simulink model "ICL2L"  (R2021a)
settings: Solver=ode1  StartTime=0.0  StopTime=30.0  FixedStep=P.ts  RelTol=1e-3  EnableMultiTasking=on
InitFcn:
  | ICL2L_PreSim
undefined symbols (not defined in the file or in its folder): P
libraries: commchan3 x2, commfilt2 x2
settings Model: Creator=rkamalapurkar  LastModifiedBy=rushik
settings SolverCC: AlgebraicLoopSolver=TrustRegion
settings DataIOCC: LimitDataPoints=on  SaveFormat=Array  SignalLoggingSaveFormat=ModelDataLogs  ReturnWorkspaceOutputs=off
settings OptimizationCC: ExpressionDepthLimit=2147483647  LifeSpan=inf
settings DebuggingCC: UnderspecifiedInitializationDetection=Classic  MergeDetectMultiDrivingBlocksExec=none  SolverPrmCheckMsg=warning  FcnCallInpInsideContextMsg=warning  StateNameClashWarn=warning  SFUnexpectedBacktrackingDiag=warning  SFNoUnconditionalDefaultTransitionDiag=warning  SFExecutionAtInitializationDiag=none  SFMachineParentedDataDiag=warning  ArithmeticOperatorsInVariantConditions=warning
settings HardwareCC: ProdBitPerPointer=32  ProdBitPerSizeT=32  ProdBitPerPtrDiffT=32  ProdLargestAtomicFloat=None  ProdIntDivRoundTo=Undefined  ProdEndianess=Unspecified  ProdWordSize=32  ProdHWDeviceType=32-bit Generic
settings ModelReferenceCC: PropagateSignalLabelsOutOfModel=off
settings SFSimCC: SimUseLocalCustomCode=off  CustomCodeUndefinedFunction=UseInterfaceOnly
settings RTWCC: RTWUseLocalCustomCode=off
settings CodeAppCC: StateflowObjectComments=on
settings GRTTargetCC: TargetLangStandard=C89/C90 (ANSI)  CombineOutputUpdateFcns=off  GRTInterface=on
settings ConfigComp: CovMetricSettings=dw  CovSaveCumulativeToWorkspaceVar=on  CovSaveSingleToWorkspaceVar=on  CovExternalEMLEnable=off  CovSFcnEnable=off

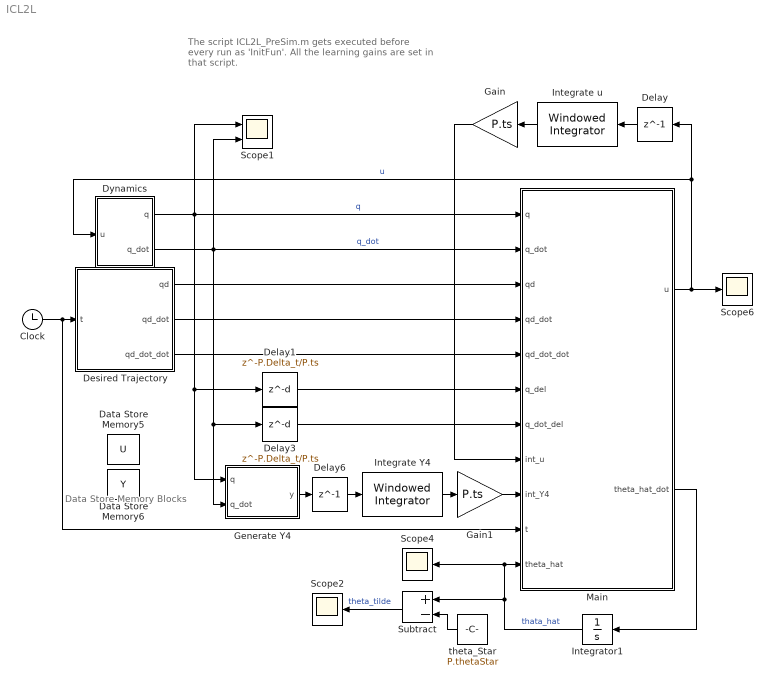
== system ICL2L ==
  note: Data Store Memory Blocks
  note: The script ICL2L_PreSim.m gets executed before every run as 'InitFun'. All the learning gains are set in that script.
  Clock : Clock
  Data Store Memory5 : DataStoreMemory  DataStoreName=U  InitialValue=zeros(P.n*P.N,1)  ShowAdditionalParam=off  OutDataTypeStr=double
  Data Store Memory6 : DataStoreMemory  DataStoreName=Y  InitialValue=zeros(P.n*P.N,P.L)  ShowAdditionalParam=off  OutDataTypeStr=double
  Delay : Delay  DelayLength=1
  Delay1 : Delay  DelayLength=P.Delta_t/P.ts  InitialCondition=0
  Delay3 : Delay  DelayLength=P.Delta_t/P.ts  InitialCondition=0
  Delay6 : Delay  DelayLength=1
  Desired Trajectory : MATLAB Function  TreatAsAtomicUnit=on
  Dynamics : Subsystem
  Gain : Gain  Gain=P.ts
  Gain1 : Gain  Gain=P.ts
  Generate Y4 : MATLAB Function  TreatAsAtomicUnit=on
  Integrate Y4 : commfilt2/Windowed Integrator  integperiod=P.Delta_t/P.ts  roundingMode=Floor  overflowMode=off  coeffDataTypeStr=Inherit: Same word length as input  coeffMin=[]  coeffMax=[]  coeffLastDataTypeStr=Inherit: Same word length as input  accumDataTypeStr=Inherit: Same as product output  accumLastDataTypeStr=Inherit: Same as product output  outputDataTypeStr=Inherit: Same as accumulator  outputMin=[]  outputMax=[]  outputLastDataTypeStr=Inherit: Same as accumulator
      settings: SourceProductBaseCode=CM
  Integrate u : commfilt2/Windowed Integrator  integperiod=P.Delta_t/P.ts  roundingMode=Floor  overflowMode=off  coeffDataTypeStr=Inherit: Same word length as input  coeffMin=[]  coeffMax=[]  coeffLastDataTypeStr=Inherit: Same word length as input  accumDataTypeStr=Inherit: Same as product output  accumLastDataTypeStr=Inherit: Same as product output  outputDataTypeStr=Inherit: Same as accumulator  outputMin=[]  outputMax=[]  outputLastDataTypeStr=Inherit: Same as accumulator
      settings: SourceProductBaseCode=CM
  Integrator1 : Integrator  InitialCondition=P.theta0
  Main : MATLAB Function  TreatAsAtomicUnit=on
  Scope1 : Scope  NumInputPorts=2
  Scope2 : Scope
  Scope4 : Scope
  Scope6 : Scope
  Subtract : Sum  Inputs=+-
  theta_Star : Constant  Value=P.thetaStar
  wires:
  Clock/1 -> Main/10(t), Desired Trajectory/1(t)
  Main/2(theta_hat_dot) -> Integrator1/1
  Integrator1/1 -> Scope4/1, Main/11(theta_hat), Subtract/1  "thata_hat"
  Dynamics/1(q) -> Scope1/1, Generate Y4/1(q), Delay1/1, Main/1(q)  "q"
  Main/1(u) -> Delay/1, Dynamics/1(u), Scope6/1  "u"
  Desired Trajectory/1(qd) -> Main/3(qd)
  Desired Trajectory/2(qd_dot) -> Main/4(qd_dot)
  Desired Trajectory/3(qd_dot_dot) -> Main/5(qd_dot_dot)
  Dynamics/2(q_dot) -> Scope1/2, Main/2(q_dot), Generate Y4/2(q_dot), Delay3/1  "q_dot"
  Delay3/1 -> Main/7(q_dot_del)
  Delay1/1 -> Main/6(q_del)
  Integrate u/1 -> Gain/1
  Gain/1 -> Main/8(int_u)
  Delay/1 -> Integrate u/1
  Integrate Y4/1 -> Gain1/1
  Gain1/1 -> Main/9(int_Y4)
  Generate Y4/1(y) -> Delay6/1
  Delay6/1 -> Integrate Y4/1
  Subtract/1 -> Scope2/1  "theta_tilde"
  theta_Star/1 -> Subtract/2

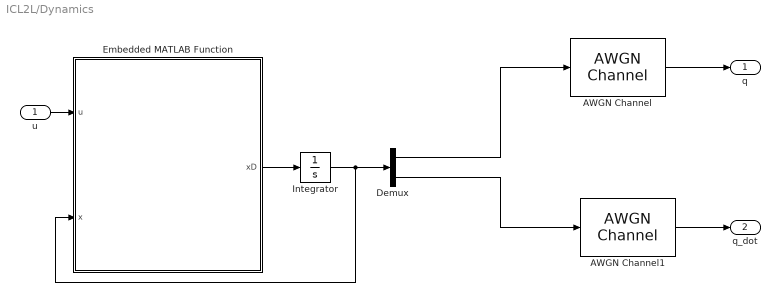
== system ICL2L/Dynamics ==
  u : Inport
  AWGN Channel : commchan3/AWGN Channel  InputProcessing=Columns as channels (frame based)  seed=67  noiseMode=Variance from mask  EbNodB=10  EsNodB=10  SNRdB=10  bitsPerSym=1  Ps=1  Tsym=1  variance=0.001
  AWGN Channel1 : commchan3/AWGN Channel  InputProcessing=Columns as channels (frame based)  seed=67  noiseMode=Variance from mask  EbNodB=10  EsNodB=10  SNRdB=10  bitsPerSym=1  Ps=1  Tsym=1  variance=0.01
  Demux : Demux  Outputs=2
  Embedded MATLAB Function : MATLAB Function  TreatAsAtomicUnit=on
  Integrator : Integrator  InitialCondition=P.x0
  q : Outport
  q_dot : Outport  Port=2
  wires:
  Integrator/1 -> Demux/1, Embedded MATLAB Function/2(x)
  Embedded MATLAB Function/1(xD) -> Integrator/1
  u/1 -> Embedded MATLAB Function/1(u)
  Demux/1 -> AWGN Channel/1
  Demux/2 -> AWGN Channel1/1
  AWGN Channel/1 -> q/1
  AWGN Channel1/1 -> q_dot/1

== matlab function ICL2L/Dynamics/Embedded MATLAB Function ==
  data: u input size=[P.n 1]; xD output size=[2*P.n 1]; x input size=[2*P.n 1]
function xD = fcn(u,x)

p1 = 3.473;
p2 = .196;
p3 = .242;
fd1 = 5.3;
fd2 = 1.1;
fs1 = 8.45;
fs2 = 2.35;

Minv = (1/(p2^2 - p1*p2 + p3^2*cos(x(2))^2))*...
       [-p2               p2+p3*cos(x(2))  ;...
         p2+p3*cos(x(2)) -p1-2*p3*cos(x(2))];

Vm = [-p3*sin(x(2))*x(4) -p3*sin(x(2))*(x(3)+x(4));
       p3*sin(x(2))*x(3)  0                      ];
Fd = diag([fd1,fd2]);
Fs = [fs1*tanh(1*x(3));fs2*tanh(1*x(4))];
f = [x(3); x(4); Minv*((-Vm - Fd)*[x(3); x(4)]-Fs)];
g = [0 0; 0 0; Minv]; 

xD = f+g*u;

== matlab function ICL2L/Generate Y4 ==
  data: q input size=[P.n 1]; y output size=[P.n P.L]; q_dot input size=[P.n 1]
function y = Y4(q,q_dot)
    y = Y4(q,q_dot);
end

== matlab function ICL2L/Desired Trajectory ==
  data: t input; qd output; qd_dot output; qd_dot_dot output
function [qd,qd_dot,qd_dot_dot] = desiredTrajectory(t)
    [qd,qd_dot,qd_dot_dot] = desiredTraj(t);
end

== matlab function ICL2L/Main ==
  settings: updateMethod=DISCRETE
  data: u output; q input size=[P.n 1]; q_dot input size=[P.n 1]; qd input; qd_dot input; qd_dot_dot input; q_del input; q_dot_del input; int_u input; int_Y4 input; t input; theta_hat input; theta_hat_dot output; U data_store_memory; P parameter; Y data_store_memory
function [u,theta_hat_dot] =...
    ICLControl(q,q_dot,qd,qd_dot,qd_dot_dot,q_del,q_dot_del,...
    int_u,int_Y4,t,theta_hat,P)
%#codegen
% This simulink block implements integral-concurrent-learning based system
% identification and adaptive control

global Y; % Data store memory for storing the values of \mathscr{Y}
          % nN x L
global U; % Data store memory for storing the values of \mathscr{U}
          % nN x 1
          
e = qd - q;
e_dot = qd_dot - q_dot;
r = e_dot + P.alpha * e;

if t > P.Delta_t
    % eigenvalue maximization data storage
    current_sum = Y.'*Y;
    current_min = min(eig(current_sum));
    new_Y = Y3(q,q_dot,q_del,q_dot_del) + int_Y4;
    new_U = int_u;
    min_store = zeros(P.N,1);
    for i=1:P.N
        new_sum = current_sum - Y(P.n*i-1:P.n*i,:).'*Y(P.n*i-1:P.n*i,:) + new_Y.'*new_Y;
        min_store(i) = real(min(eig(new_sum)));
    end
    [new_max,index] = max(min_store);
    if new_max > current_min + P.epsilon
            Y(P.n*index-1:P.n*index,:) = new_Y;
            U(P.n*index-1:P.n*index,:) = new_U;
    end

    % Update law
    theta_hat_dot = P.Gamma*Y2(q,q_dot,qd,qd_dot,qd_dot_dot,P.alpha).'*r...
        + P.k2*P.Gamma*Y.'*(U - Y*theta_hat);
else
    theta_hat_dot = zeros(size(theta_hat));
end
% Controller
u = Y2(q,q_dot,qd,qd_dot,qd_dot_dot,P.alpha)*theta_hat + e + P.k1 * r;
end
